simulink model "mmwave_sim"  (R2025a)
settings: Solver=FixedStepDiscrete  StartTime=0.0  StopTime=10.0  FixedStep=1/8000  RelTol=1e-3
values from neighbouring files (symbols this model uses):
  tx_samples = tx_samples(:)    [create_tx_signal.m]    (also in tx_workspace.mat = [0 0 0 0 0 0 0 0 0 0 0 0 ... (23360 elements, 23360x1)])
libraries: commchan3 x1
settings Model: Creator=Subham Sarkar  LastModifiedBy=Subham Sarkar

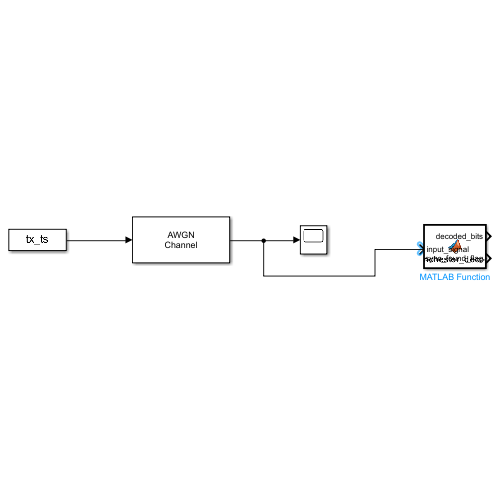
[thumbnail: Simulink's stored preview of the top-level diagram]
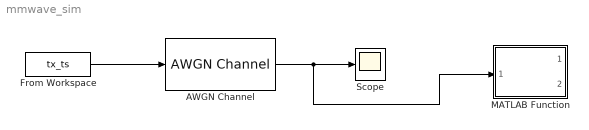
== system mmwave_sim ==
  AWGN Channel : commchan3/AWGN Channel  LegacyMode=off  NoiseMethod="Signal to noise ratio  (SNR)"  noiseMode="Signal to noise ratio  (SNR)"  EbNo=10  EsNo=10  SNR=20  BitsPerSymbol=1  SignalPower=mean(tx_samples.^2)  SpecifySymbolPeriod=off  SamplesPerSymbol=1  SymbolPeriod=1  VarianceSource=Parameter  Variance=1  RandomStream=Global stream  Seed=67  SimulateUsing=Code generation
  From Workspace : FromWorkspace  VariableName=tx_ts  SampleTime=-1  OutputAfterFinalValue=Holding final value
  MATLAB Function : MATLAB Function  TreatAsAtomicUnit=on
  Scope : Scope
      settings: TimeSpan=.1  ActiveDisplayYMinimum=-0.20543452059022688  ActiveDisplayYMaximum=0.263490220410751
  wires:
  From Workspace/1 -> AWGN Channel/1
  AWGN Channel/1 -> MATLAB Function/1(input_signal), Scope/1

== matlab function mmwave_sim/MATLAB Function ==
  data: input_signal input; decoded_bits output; sync_found_flag output
function [decoded_bits, sync_found_flag] = manchester_decoder(input_signal)
%#codegen

% Parameters
SYNC_WORD = uint32(hex2dec('AAAAAA2D'));
MAX_BITS = 1024;  % adjust buffer size
persistent bitstream bit_count in_sync

if isempty(bitstream)
    bitstream = false(1, MAX_BITS);
    bit_count = uint32(0);
    in_sync = false;
end

decoded_bits = false(1, MAX_BITS);
sync_found_flag = false;

% Step 1: Manchester pair decoding
persistent man_buf man_cnt
if isempty(man_buf)
    man_buf = false(1,2);
    man_cnt = uint8(0);
end

for k = 1:length(input_signal)
    % Accumulate pairs
    man_cnt = man_cnt + 1;
    man_buf(man_cnt) = input_signal(k);

    if man_cnt == 2
        man_cnt = uint8(0);

        % Decode valid pairs
        if man_buf(1)==1 && man_buf(2)==0
            bit_val = true;
        elseif man_buf(1)==0 && man_buf(2)==1
            bit_val = false;
        else
            % invalid pair → skip
            continue;
        end

        % Shift register for sync detection
        bit_count = bit_count + 1;
        if bit_count > MAX_BITS
            bit_count = uint32(1);
        end
        bitstream(bit_count) = bit_val;

        % Convert last 32 bits into integer
        if bit_count >= 32
            word_val = uint32(0);
            for i = 0:31
                word_val = bitor(word_val, bitshift(uint32(bitstream(bit_count - i)), i));
            end

            % Sync detection
            if ~in_sync && word_val == SYNC_WORD
                in_sync = true;
                sync_found_flag = true;
                bit_count = uint32(0); % reset counter to start fresh
            end
        end

        % If in sync → output decoded bits
        if in_sync
            decoded_bits(bit_count) = bit_val;
        end
    end
end
